simulink library "atc"  (Simulink 8.1)
settings: Solver=ode45  StartTime=0.0  StopTime=10.0  RelTol=1e-3
undefined symbols (not defined in the file): AJUD_TTCMap_X_mps, AJUD_TTCMap_Y_mps2, KJUD_AEBActDriverDelay_ms, KJUD_AEBAggrDriverDelay_ms, KJUD_AEBConsDec_mps2, KJUD_AutoBrakingDelay_ms, MJUD_TTCMap_ms, TRUE, ZERO_FLOAT
settings Model: Creator=AT015086  LastModifiedBy=tescamilla

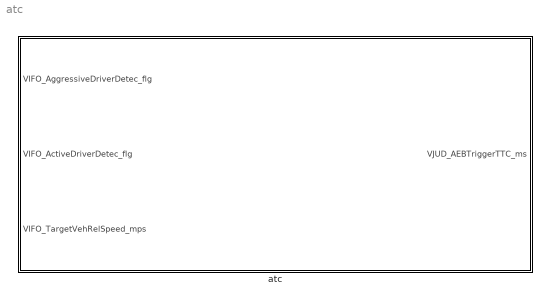
== system atc ==
  "atc " : Subsystem

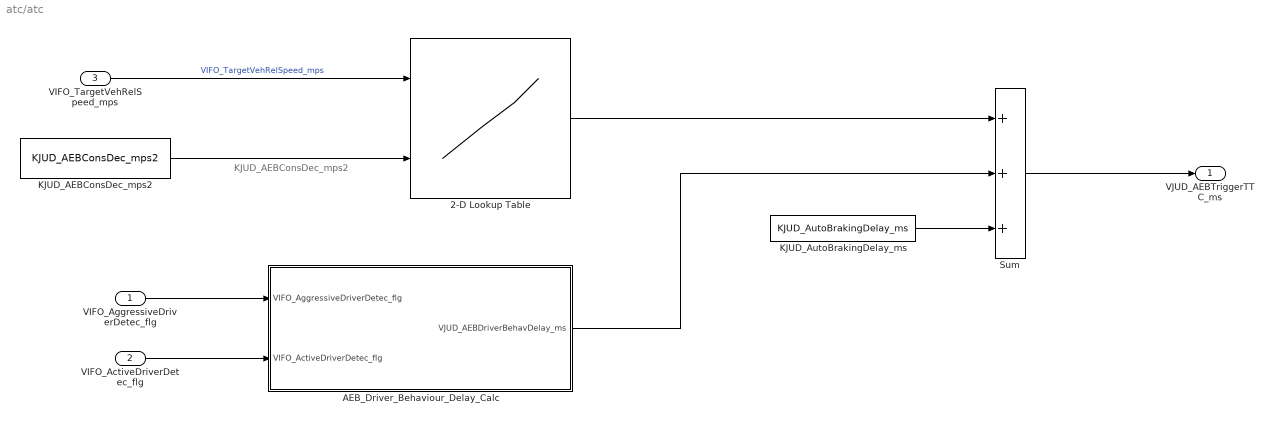
== system atc/atc  ==
  note: KJUD_AEBConsDec_mps2
  VIFO_AggressiveDriverDetec_flg : Inport
  VIFO_ActiveDriverDetec_flg : Inport  Port=2
  VIFO_TargetVehRelSpeed_mps : Inport  Port=3
  2-D Lookup Table : Lookup_n-D  BreakpointsForDimension1=AJUD_TTCMap_X_mps  BreakpointsForDimension2=AJUD_TTCMap_Y_mps2  Table=MJUD_TTCMap_ms  RndMeth=Simplest  InputSameDT=on
  AEB_Driver_Behaviour_Delay_Calc : Subsystem
  KJUD_AEBConsDec_mps2 : Constant  Value=KJUD_AEBConsDec_mps2
  KJUD_AutoBrakingDelay_ms : Constant  Value=KJUD_AutoBrakingDelay_ms
  Sum : Sum  Inputs=+++
  VJUD_AEBTriggerTTC_ms : Outport
  wires:
  VIFO_AggressiveDriverDetec_flg/1 -> AEB_Driver_Behaviour_Delay_Calc/1(VIFO_AggressiveDriverDetec_flg)
  VIFO_ActiveDriverDetec_flg/1 -> AEB_Driver_Behaviour_Delay_Calc/2(VIFO_ActiveDriverDetec_flg)
  AEB_Driver_Behaviour_Delay_Calc/1(VJUD_AEBDriverBehavDelay_ms) -> Sum/2
  KJUD_AutoBrakingDelay_ms/1 -> Sum/3
  Sum/1 -> VJUD_AEBTriggerTTC_ms/1
  VIFO_TargetVehRelSpeed_mps/1 -> 2-D Lookup Table/1  "VIFO_TargetVehRelSpeed_mps"
  KJUD_AEBConsDec_mps2/1 -> 2-D Lookup Table/2
  2-D Lookup Table/1 -> Sum/1

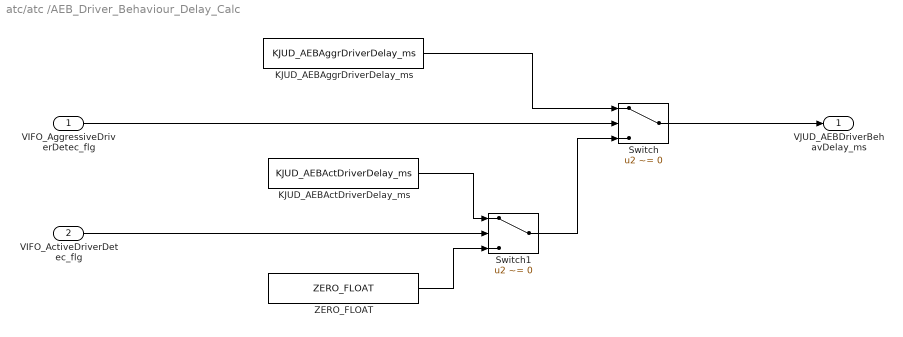
== system atc/atc /AEB_Driver_Behaviour_Delay_Calc ==
  VIFO_AggressiveDriverDetec_flg : Inport
  VIFO_ActiveDriverDetec_flg : Inport  Port=2
  KJUD_AEBActDriverDelay_ms : Constant  Value=KJUD_AEBActDriverDelay_ms
  KJUD_AEBAggrDriverDelay_ms : Constant  Value=KJUD_AEBAggrDriverDelay_ms
  Switch : Switch  Criteria=u2 ~= 0  Threshold=TRUE
  Switch1 : Switch  Criteria=u2 ~= 0  Threshold=TRUE
  ZERO_FLOAT : Constant  Value=ZERO_FLOAT
  VJUD_AEBDriverBehavDelay_ms : Outport
  wires:
  VIFO_AggressiveDriverDetec_flg/1 -> Switch/2
  KJUD_AEBAggrDriverDelay_ms/1 -> Switch/1
  Switch1/1 -> Switch/3
  VIFO_ActiveDriverDetec_flg/1 -> Switch1/2
  KJUD_AEBActDriverDelay_ms/1 -> Switch1/1
  Switch/1 -> VJUD_AEBDriverBehavDelay_ms/1
  ZERO_FLOAT/1 -> Switch1/3
